simulink model "controller_INDI"  (R2020a)
settings: Solver=FixedStepDiscrete  StartTime=0.0  StopTime=inf  FixedStep=0.01  RelTol=1e-3
PreLoadFcn:
  | %messageFolder=fullfile('..', '..', '..', '..', 'msg');
  | defineBuses_nav();
  | [constants, defaultPara]=initParametersAndConstants();
PostLoadFcn:
  | if constants.stepSize - evalin('base', get_param(bdroot, 'FixedStep')) > 10*eps('single')
  | error('inconsistent step size, check model configuration and constant settings');
  | end
settings Model: Creator=ac112430  LastModifiedBy=Bayram
settings DataIOCC: ReturnWorkspaceOutputs=off
settings OptimizationCC: DefaultParameterBehavior=Inlined  DefaultUnderspecifiedDataType=single  PassReuseOutputArgsAs=Individual arguments  EfficientTunableParamExpr=on
settings DebuggingCC: ParameterPrecisionLossMsg=none  ParameterTunabilityLossMsg=error  ArithmeticOperatorsInVariantConditions=warning
settings HardwareCC: ProdBitPerPointer=32  ProdBitPerSizeT=32  ProdBitPerPtrDiffT=32  ProdLargestAtomicInteger=Long  ProdLargestAtomicFloat=Double  ProdIntDivRoundTo=Undefined  ProdWordSize=32  ProdLongLongMode=on  ProdHWDeviceType=ARM Compatible->ARM Cortex
settings ModelReferenceCC: ModelReferenceNumInstancesAllowed=Single  PropagateSignalLabelsOutOfModel=off
settings SFSimCC: SimUseLocalCustomCode=off  MATLABDynamicMemAlloc=off  CustomCodeUndefinedFunction=UseInterfaceOnly
settings RTWCC: SystemTargetFile=ert.tlc  GenCodeOnly=on  TemplateMakefile=ert_default_tmf  RTWUseLocalCustomCode=off  BuildConfiguration=Faster Runs  IncludeHyperlinkInReport=on
settings CodeAppCC: IgnoreCustomStorageClasses=off  MaxIdLength=51  StateflowObjectComments=on
settings ERTTargetCC: TargetLangStandard=C99 (ISO)  GenerateSampleERTMain=on  SupportComplex=off  SupportVariableSizeSignals=on  InlinedParameterPlacement=NonHierarchical  ERTCustomFileTemplate=example_file_process.tlc  ConvertIfToSwitch=off  SuppressUnreachableDefaultCases=off
settings SimscapeCC: SimscapeNormalizeSystem=off

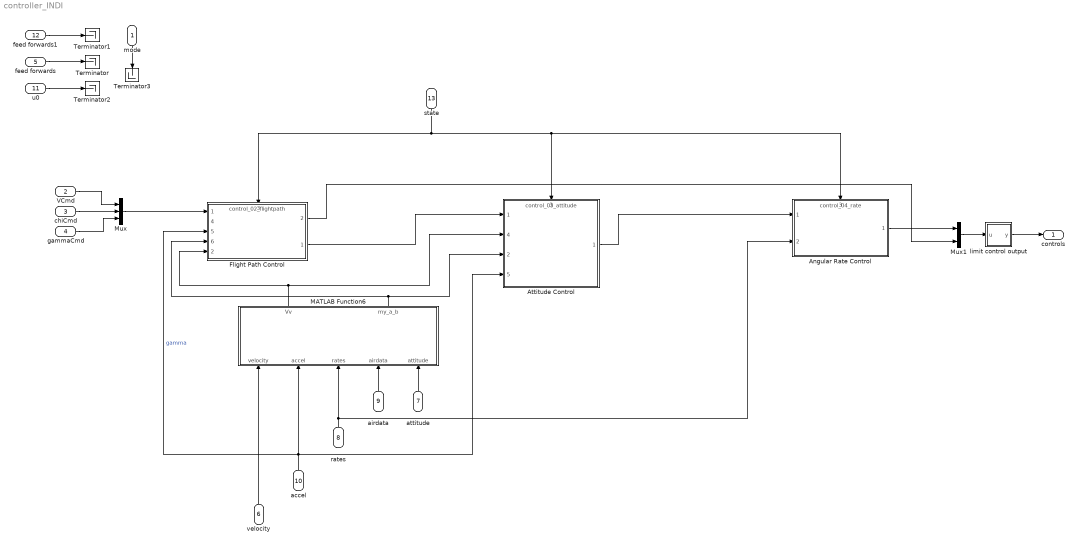
== system controller_INDI ==
  mode : Inport  OutDataTypeStr=int8
  VCmd : Inport  Port=2
  chiCmd : Inport  Port=3  PortDimensions=1
  gammaCmd : Inport  Port=4
  feed forwards : Inport  Port=5  OutDataTypeStr=Bus: ifr_ffw
  velocity : Inport  Port=6  OutDataTypeStr=single  PortDimensions=3
  attitude : Inport  Port=7  OutDataTypeStr=single  PortDimensions=3
  rates : Inport  Port=8  OutDataTypeStr=single  PortDimensions=3
  airdata : Inport  Port=9  OutDataTypeStr=single  PortDimensions=3
  accel : Inport  Port=10  OutDataTypeStr=single  PortDimensions=3
  u0 : Inport  Port=11  PortDimensions=4
  feed forwards1 : Inport  Port=12  OutDataTypeStr=Bus: parameterBus
  state : Inport  Port=13  OutDataTypeStr=Bus:fmBus
  Angular Rate Control : ModelReference  ModelNameDialog=control_04_rate.slx  SimulationMode=Normal  ModelReferenceVersion=1.15
      settings: PortSchema="{\"entries\":[{\"content\":{\"sides\":[{\"content\":{\"connectorIds\":[\"In1\",\"In2\"]},\"type\":\"ConnectorPlacement.EquallySpacedRectSide\",\"uuid\":\"dd2c7c5a-edfe-426a-90ae-4f5baec66ccc\"},{\"content\":{\"connectorIds\":[\"Out1\"],\"side\":\"RIGHT\"},\"type\":\"ConnectorPlacement.EquallySpacedRectSide\",\"uuid\":\"af81ca18-9d5a-4987-857f-5f0368661d9e\"},{\"content\":{\"connectorIds\":[\"In3\"],\"side\":\"TOP\"},\"type\":\"ConnectorPlacement.EquallySpacedRectSide\",\"uuid\":\"20a506a6-18a1-43c4-bef4-b4d77bee7dce\"}]},\"type\":\"ConnectorPlacement.EquallySpacedConnector\",\"uuid\":\"77a54400-1996-4d7f-8b83-449602bf7bcd\"}],\"packageUris\":[\"http://schema.mathworks.com/mf0/Connector/19700101\"],\"version\":\"1.0\"}"
  Attitude Control : ModelReference  ModelNameDialog=control_03_attitude.slx  SimulationMode=Normal  ModelReferenceVersion=1.33
      settings: PortSchema="{\"entries\":[{\"content\":{\"sides\":[{\"content\":{\"connectorIds\":[\"In1\",\"In4\",\"In2\",\"In5\"]},\"type\":\"ConnectorPlacement.EquallySpacedRectSide\",\"uuid\":\"dd2c7c5a-edfe-426a-90ae-4f5baec66ccc\"},{\"content\":{\"connectorIds\":[\"Out1\"],\"side\":\"RIGHT\"},\"type\":\"ConnectorPlacement.EquallySpacedRectSide\",\"uuid\":\"af81ca18-9d5a-4987-857f-5f0368661d9e\"},{\"content\":{\"connectorIds\":[\"In3\"],\"side\":\"TOP\"},\"type\":\"ConnectorPlacement.EquallySpacedRectSide\",\"uuid\":\"20a506a6-18a1-43c4-bef4-b4d77bee7dce\"}]},\"type\":\"ConnectorPlacement.EquallySpacedConnector\",\"uuid\":\"77a54400-1996-4d7f-8b83-449602bf7bcd\"}],\"packageUris\":[\"http://schema.mathworks.com/mf0/Connector/19700101\"],\"version\":\"1.0\"}"
  Flight Path Control : ModelReference  ModelNameDialog=control_02_flightpath.slx  SimulationMode=Normal  ModelReferenceVersion=1.28
      settings: PortSchema="{\"entries\":[{\"content\":{\"sides\":[{\"content\":{\"connectorIds\":[\"In1\",\"In4\",\"In5\",\"In6\",\"In2\"]},\"type\":\"ConnectorPlacement.EquallySpacedRectSide\",\"uuid\":\"c7a4ac12-8eb1-424c-9bb9-4041991d3b4d\"},{\"content\":{\"connectorIds\":[\"Out2\",\"Out1\"],\"side\":\"RIGHT\"},\"type\":\"ConnectorPlacement.EquallySpacedRectSide\",\"uuid\":\"fa6afd35-1d6d-44c9-b1b5-699b2715d7c1\"},{\"content\":{\"connectorIds\":[\"In3\"],\"side\":\"TOP\"},\"type\":\"ConnectorPlacement.EquallySpacedRectSide\",\"uuid\":\"2ca18965-e8c5-4f7d-b70c-ed373b124c43\"}]},\"type\":\"ConnectorPlacement.EquallySpacedConnector\",\"uuid\":\"67ae7afc-1252-4043-bc81-bfb0d91c1751\"}],\"packageUris\":[\"http://schema.mathworks.com/mf0/Connector/19700101\"],\"version\":\"1.0\"}"
  MATLAB Function6 : MATLAB Function  TreatAsAtomicUnit=on
  Mux : Mux  Inputs=3
  Mux1 : Mux  Inputs=2
  Terminator{,1..3} (4 alike) : Terminator
  limit control output : MATLAB Function  TreatAsAtomicUnit=on
  controls : Outport  OutDataTypeStr=double  VectorParamsAs1DForOutWhenUnconnected=off
  wires:
  Mux/1 -> Flight Path Control/1
  Flight Path Control/1 -> Attitude Control/1
  Attitude Control/1 -> Angular Rate Control/1
  feed forwards1/1 -> Terminator1/1
  feed forwards/1 -> Terminator/1
  velocity/1 -> MATLAB Function6/1(velocity)
  accel/1 -> MATLAB Function6/2(accel), Attitude Control/5, Flight Path Control/5  "gamma"
  rates/1 -> MATLAB Function6/3(rates), Angular Rate Control/2
  airdata/1 -> MATLAB Function6/4(airdata)
  attitude/1 -> MATLAB Function6/5(attitude)
  Flight Path Control/2 -> Mux1/2
  VCmd/1 -> Mux/1
  chiCmd/1 -> Mux/2
  gammaCmd/1 -> Mux/3
  MATLAB Function6/2(my_a_b) -> Flight Path Control/6, Attitude Control/2
  state/1 -> Angular Rate Control/3, Attitude Control/3, Flight Path Control/3
  Angular Rate Control/1 -> Mux1/1
  Mux1/1 -> limit control output/1(u)
  u0/1 -> Terminator2/1
  mode/1 -> Terminator3/1
  limit control output/1(y) -> controls/1
  MATLAB Function6/1(Vv) -> Attitude Control/4, Flight Path Control/2

== matlab function controller_INDI/limit control output ==
  data: u input; y output double
function y = control_output_sat(u)

y = zeros(size(u));
y(:) = min(max(u(:),-1),1);

end

== matlab function controller_INDI/MATLAB Function6 ==
  data: velocity input; Vv output; my_a_b output; accel input; rates input; airdata input; attitude input
function [Vv,my_a_b] = fcn(velocity,accel,rates,airdata,attitude)
%#codegen

chi = atan2(velocity(2), velocity(1));

Zalpha = single(-155.1208);
Ybeta  = single(-  9.0732);

r    = rates(3);
beta = accel(2)/Ybeta;
p    = rates(1);
phi  = attitude(1);

gravitation = 9.81;
alpha = (accel(3)+gravitation)/Zalpha;
q     = rates(2);
V_A   = airdata(1);
gamma = asin(-velocity(3)/norm(velocity));

Vv = [V_A; chi; gamma];
my_a_b = [0; alpha; beta];
